simulink model "Static_CDPR_V1"  (R2023b)
settings: Solver=FixedStepAuto  StartTime=0.0  StopTime=12  FixedStep=0.001  RelTol=1e-3
values from neighbouring files (symbols this model uses):
  qi = R\l0    [Initialisation.m]
  R = (sqrt(0.08^2 + 0.005^2/(2*pi))/25)    [DynModel_q.m]    (also in Initialisation.m = (sqrt(0.08^2 + 0.005^2/(2*pi))/25)   * eye(8); Rot.m = Rz * Ry * Rx; Rz.m = [cos(theta) -sin(theta) 0)
  tau_ci = quadprog(H, f, [], [], Aeq, beq, 50*ones(8,1), 5000*ones(8,1))    [Initialisation.m]    (also in TDA.m = u(13:20))
  Xi = [0, 0.0, 2.2, 0, 0, 0]'    [Initialisation.m]
settings Model: Creator=abellila  LastModifiedBy=abellila

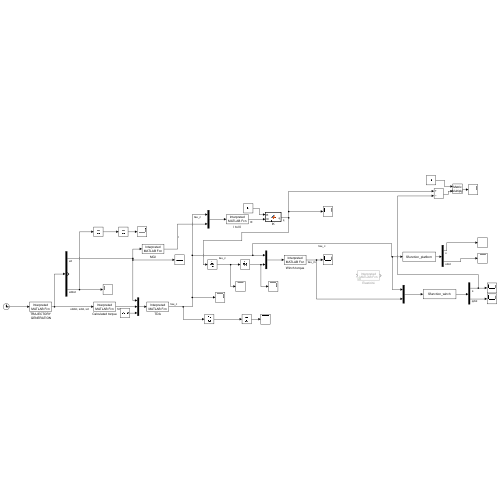
[thumbnail: Simulink's stored preview of the top-level diagram]
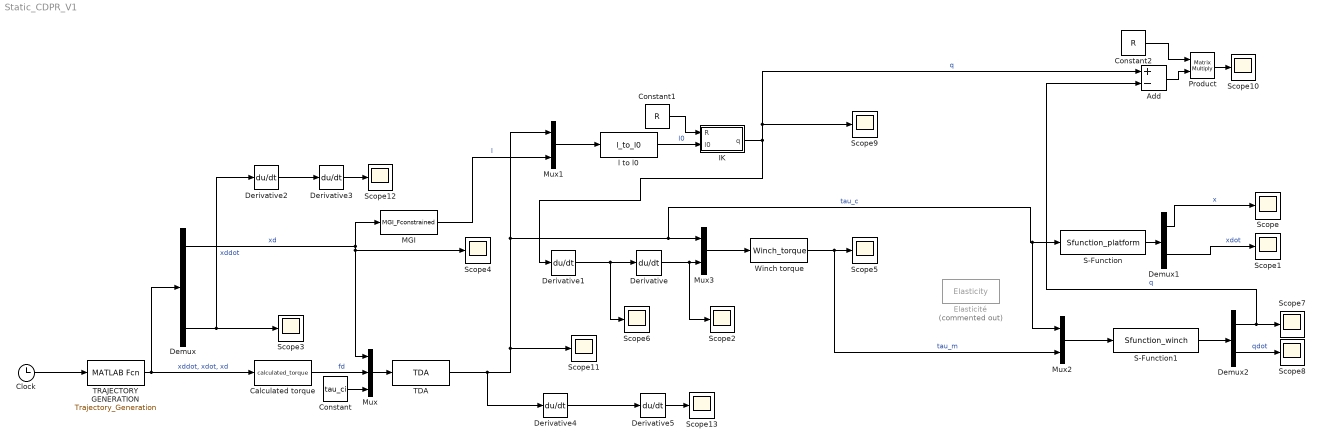
== system Static_CDPR_V1 ==
  Add : Sum  Inputs=+-
  Calculated torque : MATLABFcn  MATLABFcn=calculated_torque  Output1D=off
  Clock : Clock
  Constant : Constant  Value=tau_ci
  Constant1 : Constant  Value=R
  Constant2 : Constant  Value=R
  Demux : Demux  Outputs=3
  Demux1 : Demux  Outputs=2
  Demux2 : Demux  Outputs=2
  Derivative{,1..5} (6 alike) : Derivative
  Elasticité : MATLABFcn  Commented=on  MATLABFcn=Elasticity  OutputDimensions=8  Output1D=off
  IK : MATLAB Function  TreatAsAtomicUnit=on
  MGI : MATLABFcn  MATLABFcn=MGI_Fconstrained
  Mux : Mux  Inputs=3
  Mux1 : Mux  Inputs=2
  Mux2 : Mux  Inputs=2
  Mux3 : Mux  Inputs=2
  Product : Product  Multiplication=Matrix(*)
  S-Function : S-Function  FunctionName=Sfunction_platform  Parameters=[Xi;zeros(6,1)]  SFunctionDeploymentMode=off  EnableBusSupport=off
  S-Function1 : S-Function  FunctionName=Sfunction_winch  Parameters=[qi;zeros(8,1)]  SFunctionDeploymentMode=off  EnableBusSupport=off
  Scope{,1..13} (14 alike) : Scope
  TDA : MATLABFcn  MATLABFcn=TDA  OutputDimensions=8  Output1D=off
  TRAJECTORY GENERATION : MATLABFcn  MATLABFcn=Trajectory_Generation  Output1D=off
  Winch torque : MATLABFcn  MATLABFcn=Winch_torque
  l to l0 : MATLABFcn  MATLABFcn=l_to_l0  OutputDimensions=8  OutputSignalType=real  Output1D=off
  wires:
  Clock/1 -> TRAJECTORY GENERATION/1
  TRAJECTORY GENERATION/1 -> Calculated torque/1, Demux/1  "xddot, xdot, xd"
  Demux/1 -> Mux/1, Scope4/1, MGI/1  "xd"
  Mux/1 -> TDA/1
  TDA/1 -> Derivative4/1, Scope11/1, Mux1/1, Mux2/1, S-Function/1, Mux3/1  "tau_c"
  S-Function/1 -> Demux1/1
  Demux1/1 -> Scope/1  "x"
  Demux1/2 -> Scope1/1  "xdot"
  Constant/1 -> Mux/3
  Calculated torque/1 -> Mux/2  "fd"
  Demux/3 -> Derivative2/1, Scope3/1  "xddot"
  MGI/1 -> Mux1/2  "l"
  Mux1/1 -> l to l0/1
  Mux3/1 -> Winch torque/1
  IK/1(q) -> Derivative1/1, Add/1, Scope9/1  "q"
  l to l0/1 -> IK/2(l0)  "l0"
  Constant1/1 -> IK/1(R)
  Winch torque/1 -> Mux2/2, Scope5/1  "tau_m"
  Mux2/1 -> S-Function1/1
  Demux2/1 -> Add/2, Scope7/1  "q"
  Demux2/2 -> Scope8/1  "qdot"
  S-Function1/1 -> Demux2/1
  Add/1 -> Product/2
  Constant2/1 -> Product/1
  Product/1 -> Scope10/1
  Derivative1/1 -> Derivative/1, Scope6/1
  Derivative/1 -> Scope2/1, Mux3/2
  Derivative2/1 -> Derivative3/1
  Derivative3/1 -> Scope12/1
  Derivative4/1 -> Derivative5/1
  Derivative5/1 -> Scope13/1

== matlab function Static_CDPR_V1/IK ==
  data: R input; q output; l0 input
function q = fcn(R, l0)

q = R\l0;
